simulink model "backstep"  (Simulink 8.4)
settings: Solver=ode45  StartTime=0.0  StopTime=100  RelTol=1e-5
settings Model: Creator=jhung  LastModifiedBy=johnhung  ExtModeAutoUpdateStatusClock=off
settings DataIOCC: LimitDataPoints=off  SaveOutput=off  SaveState=on  StateSaveName=x  TimeSaveName=t  SignalLoggingName=sigsOut
settings OptimizationCC: ExpressionDepthLimit=128
settings DebuggingCC: SaveWithParameterizedLinksMsg=none  SignalResolutionControl=TryResolveAllWithWarning  SolverPrmCheckMsg=none  MultiTaskDSMMsg=warning  MultiTaskCondExecSysMsg=none  FcnCallInpInsideContextMsg=EnableAllAsError  StateNameClashWarn=none
settings HardwareCC: TargetUnknown=on
settings RTWCC: IncludeERTFirstTime=on

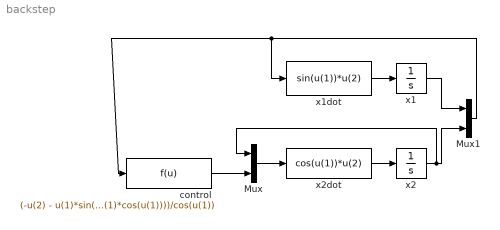
== system backstep ==
  Mux : Mux  Inputs=2
  Mux1 : Mux  Inputs=2
  control : Fcn  Expr=(-u(2) - u(1)*sin(u(1)) - sin(u(1))*u(2)*(sin(u(1))+u(1)*cos(u(1))))/cos(u(1))
  x1 : Integrator  InitialCondition=1
  x1dot : Fcn  Expr=sin(u(1))*u(2)
  x2 : Integrator  InitialCondition=1
  x2dot : Fcn  Expr=cos(u(1))*u(2)
  wires:
  x2dot/1 -> x2/1
  x1dot/1 -> x1/1
  x1/1 -> Mux1/1
  x2/1 -> Mux1/2, Mux/1
  Mux1/1 -> x1dot/1, control/1
  Mux/1 -> x2dot/1
  control/1 -> Mux/2
